simulink model "SM_fblin_singletrack_schlacher"  (R2021a)
settings: Solver=VariableStepAuto  StartTime=0.0  StopTime=5  FixedStep=1e-6  RelTol=1e-3
PostLoadFcn:
  | clear all;
  | 
  | lf  = 0.1368;
  | lr  = 0.1232;
  | m  = 1.9;
  | mu = 0.385;
  | Cf = 50.13;
  | Cr = 122.05;
  | J = 0.029;
  | 
  | V0 = 1;
  | 
  | Ts_cont = 0.001;
  | w1_gain = 20;
  | w2_gain = 100;
undefined symbols (not defined in the file or in its folder): Ts_SM
libraries: simulink x1
settings Model: Creator=l_lan  LastModifiedBy=bascetta
settings SolverCC: MaxConsecutiveZCs=10000  MaxConsecutiveMinStep=1000
settings DataIOCC: SaveOutput=off  SignalLogging=off  DSMLogging=off  SaveTime=off  ReturnWorkspaceOutputs=off

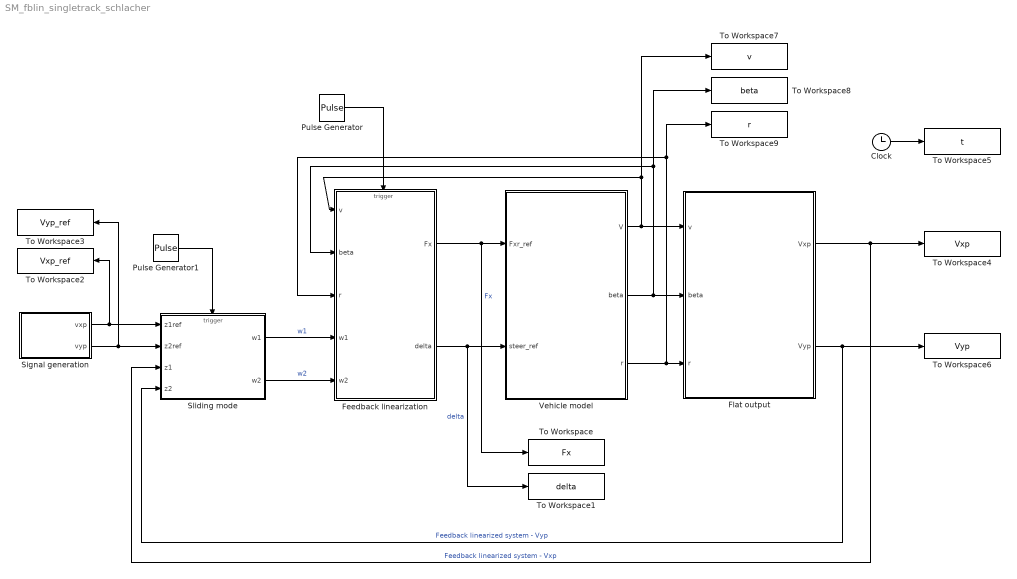
== system SM_fblin_singletrack_schlacher ==
  Clock : Clock
  Feedback linearization : Subsystem  TreatAsAtomicUnit=on
  Flat output : Subsystem
  Pulse Generator : DiscretePulseGenerator  PulseType=Time based  Period=Ts_cont  PulseWidth=50
  Pulse Generator1 : DiscretePulseGenerator  PulseType=Time based  Period=Ts_cont  PulseWidth=50
  Signal generation : Subsystem
  Sliding mode : Subsystem  TreatAsAtomicUnit=on
  To Workspace : ToWorkspace  VariableName=Fx  SampleTime=0.001
      settings: Save2DSignal=2-D array (concatenate along first dimension)
  To Workspace1 : ToWorkspace  VariableName=delta  SampleTime=0.001
      settings: Save2DSignal=2-D array (concatenate along first dimension)
  To Workspace2 : ToWorkspace  VariableName=Vxp_ref  SampleTime=0.001
      settings: Save2DSignal=2-D array (concatenate along first dimension)
  To Workspace3 : ToWorkspace  VariableName=Vyp_ref  SampleTime=0.001
      settings: Save2DSignal=2-D array (concatenate along first dimension)
  To Workspace4 : ToWorkspace  VariableName=Vxp  SampleTime=0.001
      settings: Save2DSignal=2-D array (concatenate along first dimension)
  To Workspace5 : ToWorkspace  VariableName=t  SampleTime=0.001
      settings: Save2DSignal=2-D array (concatenate along first dimension)
  To Workspace6 : ToWorkspace  VariableName=Vyp  SampleTime=0.001
      settings: Save2DSignal=2-D array (concatenate along first dimension)
  To Workspace7 : ToWorkspace  VariableName=v  SampleTime=0.001
      settings: Save2DSignal=2-D array (concatenate along first dimension)
  To Workspace8 : ToWorkspace  VariableName=beta  SampleTime=0.001
      settings: Save2DSignal=2-D array (concatenate along first dimension)
  To Workspace9 : ToWorkspace  VariableName=r  SampleTime=0.001
      settings: Save2DSignal=2-D array (concatenate along first dimension)
  Vehicle model : Subsystem
  wires:
  Vehicle model/3(r) -> Flat output/3(r), Feedback linearization/3(r), To Workspace9/1
  Flat output/2(Vyp) -> Sliding mode/4(z2), To Workspace6/1  "Feedback linearized system - Vyp"
  Flat output/1(Vxp) -> Sliding mode/3(z1), To Workspace4/1  "Feedback linearized system - Vxp"
  Clock/1 -> To Workspace5/1
  Vehicle model/2(beta) -> Flat output/2(beta), Feedback linearization/2(beta), To Workspace8/1
  Vehicle model/1(V) -> Flat output/1(v), Feedback linearization/1(v), To Workspace7/1
  Pulse Generator/1 -> Feedback linearization/Trigger
  Feedback linearization/1(Fx) -> Vehicle model/1(Fxr_ref), To Workspace/1  "Fx"
  Feedback linearization/2(delta) -> Vehicle model/2(steer_ref), To Workspace1/1  "delta"
  Signal generation/1(vxp) -> To Workspace2/1, Sliding mode/1(z1ref)
  Signal generation/2(vyp) -> To Workspace3/1, Sliding mode/2(z2ref)
  Pulse Generator1/1 -> Sliding mode/Trigger
  Sliding mode/1(w1) -> Feedback linearization/4(w1)  "w1"
  Sliding mode/2(w2) -> Feedback linearization/5(w2)  "w2"

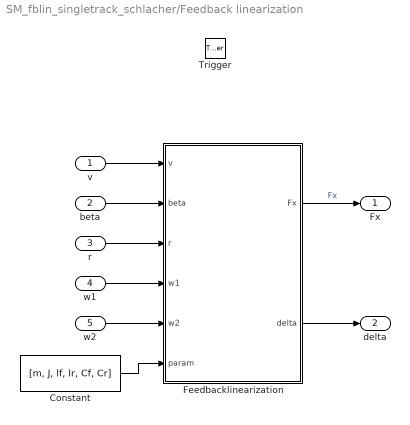
== system SM_fblin_singletrack_schlacher/Feedback linearization ==
  v : Inport
  beta : Inport  Port=2
  r : Inport  Port=3
  w1 : Inport  Port=4
  w2 : Inport  Port=5
  Trigger : TriggerPort  VariantControl=(inherit)
  Constant : Constant  Value=[m, J, lf, lr, Cf, Cr]
  Feedbacklinearization : MATLAB Function  TreatAsAtomicUnit=on
  Fx : Outport
  delta : Outport  Port=2
  wires:
  Constant/1 -> Feedbacklinearization/6(param)
  v/1 -> Feedbacklinearization/1(v)
  beta/1 -> Feedbacklinearization/2(beta)
  r/1 -> Feedbacklinearization/3(r)
  w1/1 -> Feedbacklinearization/4(w1)
  w2/1 -> Feedbacklinearization/5(w2)
  Feedbacklinearization/2(delta) -> delta/1
  Feedbacklinearization/1(Fx) -> Fx/1  "Fx"

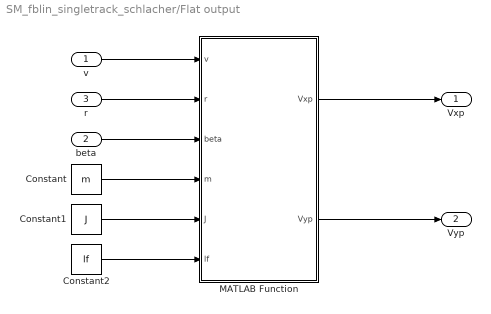
== system SM_fblin_singletrack_schlacher/Flat output ==
  v : Inport
  beta : Inport  Port=2
  r : Inport  Port=3
  Constant : Constant  Value=m
  Constant1 : Constant  Value=J
  Constant2 : Constant  Value=lf
  MATLAB Function : MATLAB Function  TreatAsAtomicUnit=on
  Vxp : Outport
  Vyp : Outport  Port=2
  wires:
  beta/1 -> MATLAB Function/3(beta)
  r/1 -> MATLAB Function/2(r)
  v/1 -> MATLAB Function/1(v)
  Constant1/1 -> MATLAB Function/5(J)
  Constant/1 -> MATLAB Function/4(m)
  Constant2/1 -> MATLAB Function/6(lf)
  MATLAB Function/2(Vyp) -> Vyp/1
  MATLAB Function/1(Vxp) -> Vxp/1

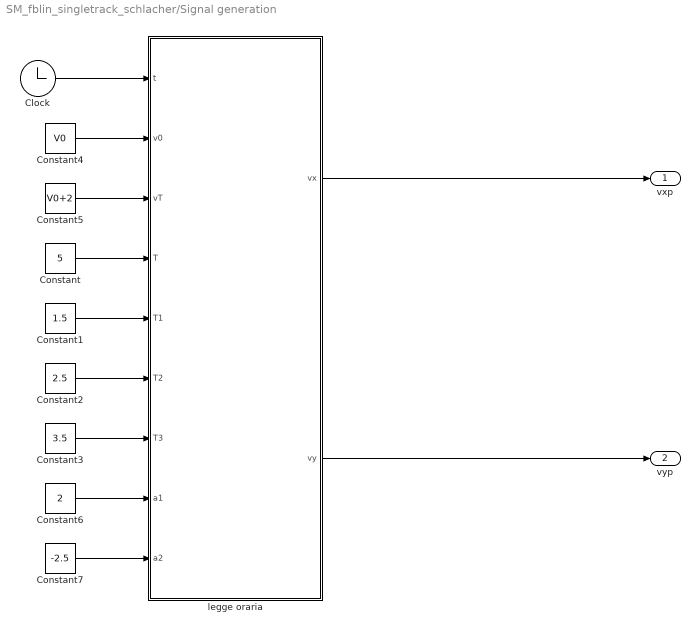
== system SM_fblin_singletrack_schlacher/Signal generation ==
  Clock : Clock
  Constant : Constant  Value=5
  Constant1 : Constant  Value=1.5
  Constant2 : Constant  Value=2.5
  Constant3 : Constant  Value=3.5
  Constant4 : Constant  Value=V0
  Constant5 : Constant  Value=V0+2
  Constant6 : Constant  Value=2
  Constant7 : Constant  Value=-2.5
  legge oraria : MATLAB Function  TreatAsAtomicUnit=on
  vxp : Outport
  vyp : Outport  Port=2
  wires:
  Clock/1 -> legge oraria/1(t)
  legge oraria/1(vx) -> vxp/1
  legge oraria/2(vy) -> vyp/1
  Constant1/1 -> legge oraria/5(T1)
  Constant/1 -> legge oraria/4(T)
  Constant2/1 -> legge oraria/6(T2)
  Constant3/1 -> legge oraria/7(T3)
  Constant4/1 -> legge oraria/2(v0)
  Constant5/1 -> legge oraria/3(vT)
  Constant6/1 -> legge oraria/8(a1)
  Constant7/1 -> legge oraria/9(a2)

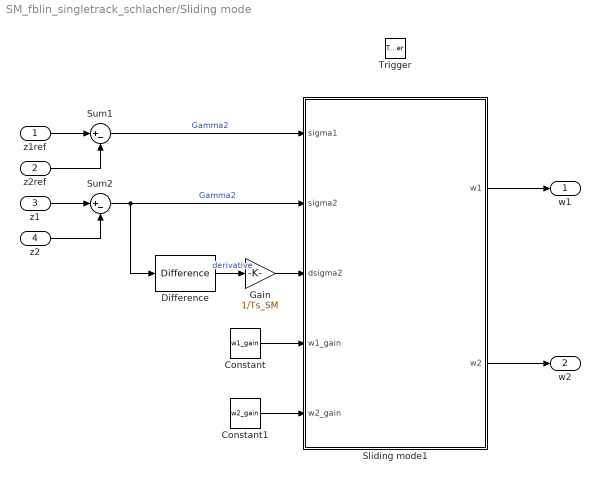
== system SM_fblin_singletrack_schlacher/Sliding mode ==
  z1ref : Inport
  z2ref : Inport  Port=2
  z1 : Inport  Port=3
  z2 : Inport  Port=4
  Trigger : TriggerPort  VariantControl=(inherit)
  Constant : Constant  Value=w1_gain
  Constant1 : Constant  Value=w2_gain
  Difference : simulink/Discrete/Difference  ICPrevInput=0.0  OutMin=[]  OutMax=[]  OutDataType=fixdt(1, 16)  OutScaling=2^-10  DoSatur=off
  Gain : Gain  Gain=1/Ts_SM
  Sliding mode1 : MATLAB Function  TreatAsAtomicUnit=on
  Sum1 : Sum  Inputs=|+-
  Sum2 : Sum  Inputs=|+-
  w1 : Outport
  w2 : Outport  Port=2
  wires:
  z1/1 -> Sum2/1
  Difference/1 -> Gain/1  "derivative"
  Constant1/1 -> Sliding mode1/5(w2_gain)
  Sum1/1 -> Sliding mode1/1(sigma1)  "Gamma2"
  z1ref/1 -> Sum1/1
  Sliding mode1/2(w2) -> w2/1
  Sum2/1 -> Difference/1, Sliding mode1/2(sigma2)  "Gamma2"
  Sliding mode1/1(w1) -> w1/1
  z2/1 -> Sum2/2
  Constant/1 -> Sliding mode1/4(w1_gain)
  z2ref/1 -> Sum1/2
  Gain/1 -> Sliding mode1/3(dsigma2)

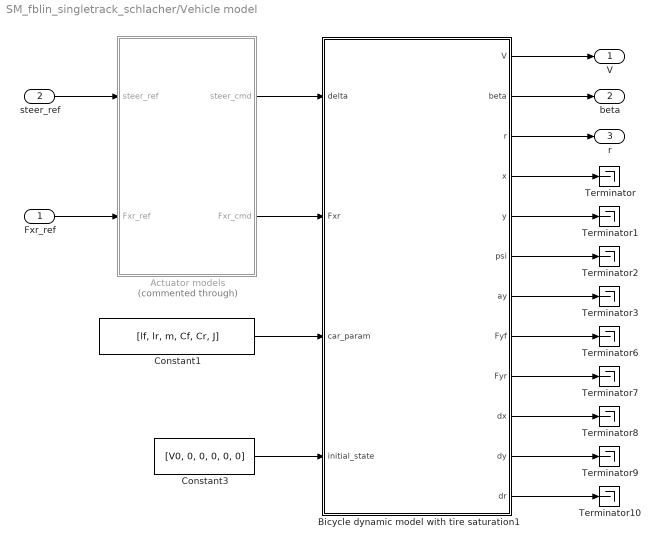
== system SM_fblin_singletrack_schlacher/Vehicle model ==
  Fxr_ref : Inport
  steer_ref : Inport  Port=2
  Actuator models : Subsystem  Commented=through  mask{mu_steer=1.0, wn_steer=87.62, csi_steer=0.75, tau_steer=0.055, steer_initial=0.0, mu_force=5.1282, wn_force=1000, csi_force=0.9, tau_force=0.0001, force_initial=0}
      mask prompts: mu_steer "Gain"; wn_steer "Natural frequency"; csi_steer "Damping"; tau_steer "Delay"; steer_initial "Initial value"; mu_force "Gain"; wn_force "Natural frequency"; csi_force "Damping"; tau_force "Delay"; force_initial "Initial value"
      mask DialogControl Container3 Prompt: Steer actuator parameters
      mask DialogControl Container4 Prompt: Speed actuator parameters
  Bicycle dynamic model with tire saturation1 : Subsystem
  Constant1 : Constant  Value=[lf, lr, m, Cf, Cr, J]
  Constant3 : Constant  Value=[V0, 0, 0, 0, 0, 0]
  Terminator{,1..3,6..10} (9 alike) : Terminator
  V : Outport
  beta : Outport  Port=2
  r : Outport  Port=3
  wires:
  Constant1/1 -> Bicycle dynamic model with tire saturation1/3(car_param)
  steer_ref/1 -> Actuator models/1(steer_ref)
  Actuator models/2(Fxr_cmd) -> Bicycle dynamic model with tire saturation1/2(Fxr)
  Fxr_ref/1 -> Actuator models/2(Fxr_ref)
  Actuator models/1(steer_cmd) -> Bicycle dynamic model with tire saturation1/1(delta)
  Constant3/1 -> Bicycle dynamic model with tire saturation1/4("initial_state ")
  Bicycle dynamic model with tire saturation1/3(r) -> r/1
  Bicycle dynamic model with tire saturation1/2(beta) -> beta/1
  Bicycle dynamic model with tire saturation1/1(V) -> V/1
  Bicycle dynamic model with tire saturation1/4(x) -> Terminator/1
  Bicycle dynamic model with tire saturation1/5(y) -> Terminator1/1
  Bicycle dynamic model with tire saturation1/6(psi) -> Terminator2/1
  Bicycle dynamic model with tire saturation1/7(ay) -> Terminator3/1
  Bicycle dynamic model with tire saturation1/8(Fyf) -> Terminator6/1
  Bicycle dynamic model with tire saturation1/9(Fyr) -> Terminator7/1
  Bicycle dynamic model with tire saturation1/10(dx) -> Terminator8/1
  Bicycle dynamic model with tire saturation1/11(dy) -> Terminator9/1
  Bicycle dynamic model with tire saturation1/12(dr) -> Terminator10/1

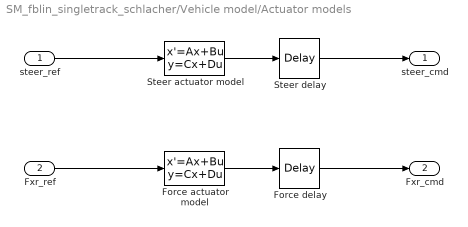
== system SM_fblin_singletrack_schlacher/Vehicle model/Actuator models ==
  steer_ref : Inport
  Fxr_ref : Inport  Port=2
  Force actuator model : StateSpace  A=[0, 1; -wn_force^2, -2*csi_force*wn_force]  B=[0; mu_force*wn_force^2]  C=[1, 0]  D=0  InitialCondition=[force_initial, 0]
  Force delay : TransportDelay  DelayTime=tau_force  InitialOutput=force_initial
  Steer actuator model : StateSpace  A=[0, 1; -wn_steer^2, -2*csi_steer*wn_steer]  B=[0; mu_steer*wn_steer^2]  C=[1, 0]  D=0  InitialCondition=[steer_initial, 0]
  Steer delay : TransportDelay  DelayTime=tau_steer  InitialOutput=steer_initial
  steer_cmd : Outport
  Fxr_cmd : Outport  Port=2
  wires:
  Fxr_ref/1 -> Force actuator model/1
  Steer actuator model/1 -> Steer delay/1
  Force actuator model/1 -> Force delay/1
  steer_ref/1 -> Steer actuator model/1
  Steer delay/1 -> steer_cmd/1
  Force delay/1 -> Fxr_cmd/1

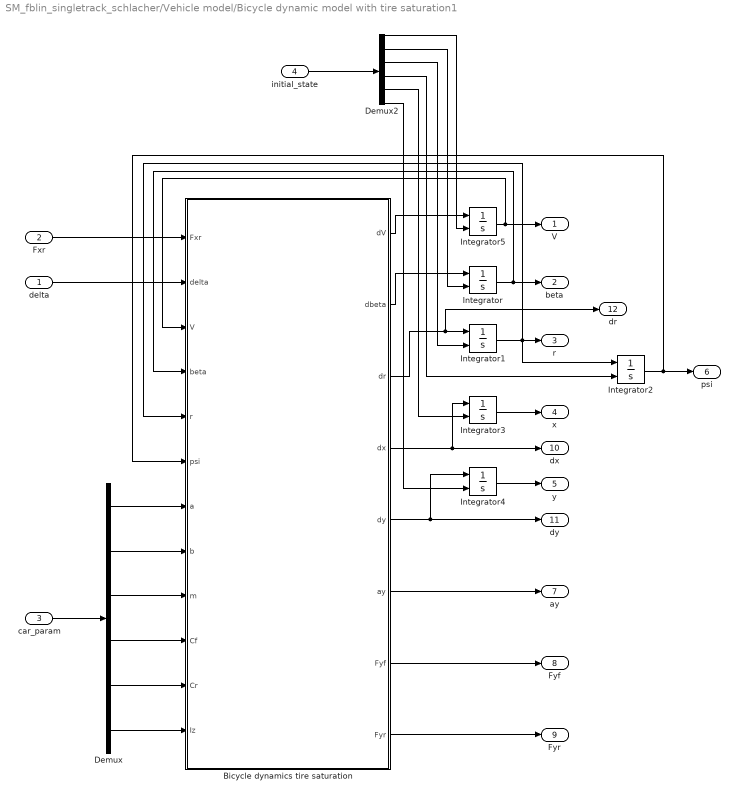
== system SM_fblin_singletrack_schlacher/Vehicle model/Bicycle dynamic model with tire saturation1 ==
  delta : Inport
  Fxr : Inport  Port=2
  car_param : Inport  Port=3
  "initial_state " : Inport  Port=4
  Bicycle dynamics tire saturation : MATLAB Function  TreatAsAtomicUnit=on
  Demux : Demux  Outputs=6
  Demux2 : Demux  Outputs=6
  Integrator{,1..5} (6 alike) : Integrator  InitialConditionSource=external
  V : Outport
  beta : Outport  Port=2
  r : Outport  Port=3
  x : Outport  Port=4
  y : Outport  Port=5
  psi : Outport  Port=6
  ay : Outport  Port=7
  Fyf : Outport  Port=8
  Fyr : Outport  Port=9
  dx : Outport  Port=10
  dy : Outport  Port=11
  dr : Outport  Port=12
  wires:
  Fxr/1 -> Bicycle dynamics tire saturation/1(Fxr)
  delta/1 -> Bicycle dynamics tire saturation/2(delta)
  Bicycle dynamics tire saturation/2(dbeta) -> Integrator/1
  Bicycle dynamics tire saturation/3(dr) -> dr/1, Integrator1/1
  Integrator/1 -> beta/1, Bicycle dynamics tire saturation/4(beta)
  Integrator1/1 -> r/1, Integrator2/1, Bicycle dynamics tire saturation/5(r)
  Bicycle dynamics tire saturation/6(ay) -> ay/1
  Bicycle dynamics tire saturation/7(Fyf) -> Fyf/1
  Bicycle dynamics tire saturation/8(Fyr) -> Fyr/1
  car_param/1 -> Demux/1
  Demux/1 -> Bicycle dynamics tire saturation/7(a)
  Demux/2 -> Bicycle dynamics tire saturation/8(b)
  Demux/3 -> Bicycle dynamics tire saturation/9(m)
  "initial_state "/1 -> Demux2/1
  Bicycle dynamics tire saturation/4(dx) -> Integrator3/1, dx/1
  Bicycle dynamics tire saturation/5(dy) -> Integrator4/1, dy/1
  Integrator3/1 -> x/1
  Integrator4/1 -> y/1
  Integrator2/1 -> Bicycle dynamics tire saturation/6(psi), psi/1
  Integrator5/1 -> V/1, Bicycle dynamics tire saturation/3(V)
  Demux2/1 -> Integrator5/2
  Bicycle dynamics tire saturation/1(dV) -> Integrator5/1
  Demux2/2 -> Integrator/2
  Demux2/3 -> Integrator1/2
  Demux2/4 -> Integrator2/2
  Demux2/5 -> Integrator3/2
  Demux2/6 -> Integrator4/2
  Demux/4 -> Bicycle dynamics tire saturation/10(Cf)
  Demux/5 -> Bicycle dynamics tire saturation/11(Cr)
  Demux/6 -> Bicycle dynamics tire saturation/12(Iz)

== matlab function SM_fblin_singletrack_schlacher/Flat output/MATLAB Function ==
  data: v input; Vxp output; r input; beta input; m input; J input; lf input; Vyp output
function [Vxp,Vyp] = z_tranform(v,r,beta,m,J,lf)

Vxp = v*cos(beta);
Vyp = v*sin(beta)-J/(m*lf)*r;

== matlab function SM_fblin_singletrack_schlacher/Vehicle model/Bicycle dynamic model with tire saturation1/Bicycle dynamics tire saturation ==
  data: dV output; dbeta output; Fxr input; dr output; dx output; dy output; delta input; V input; beta input; r input; psi input; a input; b input; m input; Cf input; Cr input; Iz input; ay output; Fyf output; Fyr output
function [dV,dbeta,dr,dx,dy,ay,Fyf,Fyr]  = bicycle_dynamics(Fxr, delta, V, beta, r, psi, a, b, m, Cf, Cr, Iz)

if (abs(V*cos(beta))<=0.01)
    Fyf = 0;
    Fyr = 0;
else
    Fyf = -Cf*((V*sin(beta)+a*r)/(V*cos(beta))-delta);
    Fyr = -Cr*(V*sin(beta)-b*r)/(V*cos(beta));
end

dV    = (Fyf*(sin(beta)-cos(beta)*delta)+Fyr*sin(beta)+Fxr*cos(beta))/m;
dbeta = (Fyf*(cos(beta)+sin(beta)*delta)+Fyr*cos(beta)-Fxr*sin(beta))/(m*V)-r;
dr    = (a*Fyf-b*Fyr)/Iz;

ay    = (sin(beta)*dV+V*(cos(beta)^2-sin(beta)^2)/cos(beta)*dbeta)+r*V*cos(beta);

R_psi = [cos(psi), -sin(psi); sin(psi), cos(psi)];
dx  = R_psi(1,1:2)*[V*cos(beta); V*sin(beta)];
dy  = R_psi(2,1:2)*[V*cos(beta); V*sin(beta)];

== matlab function SM_fblin_singletrack_schlacher/Feedback linearization/Feedbacklinearization ==
  data: v input; beta input; r input; w1 input; w2 input; Fx output; delta output; param input
function [Fx, delta] = fblin(v, beta, r, w1, w2, param)
m  = param(1);
J  = param(2);
lf = param(3);
lr = param(4);
Cf = param(5);
Cr = param(6);

l = (lf+lr)/(m*lf);
F = -(lf*v)/J*cos(beta)+(Cr*l)./(J*m*v*cos(beta))*(lf*lr*m-J);
R = (lr*v)/J*cos(beta)-(Cr*l)./(J*m*v*cos(beta))*(J+m*lr^2);
H = -r*w1+(Cr*l)./(v*cos(beta)).^2*(v*w1*sin(beta)-lr*r*w1-v^2*r*sin(beta)^2+r*v^2);
 
Fry   = Cr*(lr*r-v*sin(beta))./(v*cos(beta));        
delta = (w2-Fry*R-H)./(F*Cf)+(v*sin(beta)+lf*r)./(v*cos(beta));
Ffy   = Cf*(delta-(v*sin(beta)+lf*r)./(v*cos(beta)));     
Fx    = m*w1+Ffy*delta-v*r*m*sin(beta);

== matlab function SM_fblin_singletrack_schlacher/Signal generation/legge oraria ==
  data: t input; vx output; vy output; v0 input; vT input; T input; T1 input; T2 input; T3 input; a1 input; a2 input
function [vx,vy] = trajectory(t,v0,vT,T,T1,T2,T3,a1,a2)

vx = v0+(3*t^2*T-2*t^3)/(T^3)*(vT-v0);

if (t<=T1)
    vy = 0;
elseif (t<=T2)
    vy = -a1*((t-T1)^3)*((T2-T1)-(t-T1))^3/(T2-T1)^6;
elseif (t<=T3)
    vy = -a2*((t-T2)^3)*((T3-T2)-(t-T2))^3/(T3-T2)^6;
else
    vy = 0;
end

== matlab function SM_fblin_singletrack_schlacher/Sliding mode/Sliding mode1 ==
  data: sigma1 input; w1 output; w2 output; sigma2 input; dsigma2 input; w1_gain input; w2_gain input
function [w1,w2] = sliding_mode(sigma1,sigma2,dsigma2,w1_gain,w2_gain)

w1 = w1_gain*sign(sigma1);
w2 = w2_gain*sign(sigma2+dsigma2*abs(dsigma2)/(2*w2_gain));
